simulink model "gm_distortion"  (R2024a)
settings: Solver=VariableStepAuto  StartTime=0.0  StopTime=120  RelTol=1e-3
settings Model: Creator=EAGLEAORUS  LastModifiedBy=fermata
settings OptimizationCC: BlockReduction=off  ConditionallyExecuteInputs=off
settings DebuggingCC: InheritedTsInSrcMsg=none

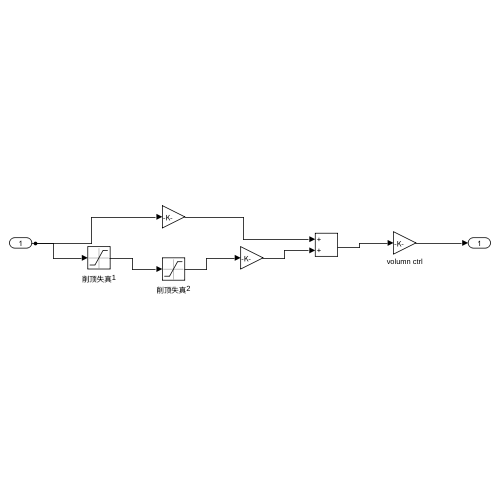
[thumbnail: Simulink's stored preview of the top-level diagram]
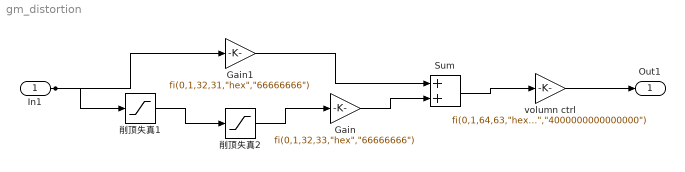
== system gm_distortion ==
  In1 : Inport  OutDataTypeStr=int32  PortDimensions=1  SampleTime=0
  Gain : Gain  Gain="fi(0,1,32,33,\"hex\",\"66666666\")"  ParamDataTypeStr=fixdt(1, 32, 33)  OutDataTypeStr=fixdt(1, 64, 33)  SampleTime=0
  Gain1 : Gain  Gain="fi(0,1,32,31,\"hex\",\"66666666\")"  ParamDataTypeStr=fixdt(1, 32, 31)  OutDataTypeStr=fixdt(1, 64, 31)  SampleTime=0
  Sum : Sum  OutDataTypeStr=fixdt(1, 64, 31)  AccumDataTypeStr=fixdt(1, 64, 31)  SampleTime=0
  volumn ctrl : Gain  Gain="fi(0,1,64,63,\"hex\",\"4000000000000000\")"  ParamDataTypeStr=fixdt(1, 64, 63)  OutDataTypeStr=int32  SaturateOnIntegerOverflow=on  SampleTime=0
  削顶失真1 : Saturate  UpperLimit="fi(0,1,32,0,\"hex\",\"00000000\")"  LowerLimit="fi(0,1,32,0,\"hex\",\"00000000\")"  SampleTime=0  OutDataTypeStr=int32
  削顶失真2 : Saturate  UpperLimit="fi(0,1,32,0,\"hex\",\"00000000\")"  LowerLimit="fi(0,1,32,0,\"hex\",\"00000000\")"  SampleTime=0  OutDataTypeStr=int32  RndMeth=Convergent
  Out1 : Outport  OutDataTypeStr=int32  SampleTime=0  VectorParamsAs1DForOutWhenUnconnected=off
  wires:
  In1/1 -> 削顶失真1/1, Gain1/1
  Gain/1 -> Sum/2
  Gain1/1 -> Sum/1
  Sum/1 -> volumn ctrl/1
  volumn ctrl/1 -> Out1/1
  削顶失真1/1 -> 削顶失真2/1
  削顶失真2/1 -> Gain/1
